simulink library "SatDyn"  (R2018a)
settings: Solver=ode45  StartTime=0.0  StopTime=10.0  RelTol=1e-3
undefined symbols (not defined in the file): ConfParam
settings Model: Creator=y.akisheva  LastModifiedBy=Cédric
settings DataIOCC: LimitDataPoints=on  SaveFormat=Array
settings OptimizationCC: BlockReduction=off  BooleanDataType=off  LifeSpan=inf
settings DebuggingCC: SaveWithParameterizedLinksMsg=none  UnderspecifiedInitializationDetection=Classic  MergeDetectMultiDrivingBlocksExec=none  SignalResolutionControl=TryResolveAllWithWarning  SFUnexpectedBacktrackingDiag=warning  SFNoUnconditionalDefaultTransitionDiag=warning  SFExecutionAtInitializationDiag=none
settings HardwareCC: ProdBitPerPointer=32  ProdBitPerSizeT=32  ProdBitPerPtrDiffT=32  ProdLargestAtomicFloat=None  ProdIntDivRoundTo=Undefined  ProdEndianess=Unspecified  ProdWordSize=32  ProdHWDeviceType=32-bit Generic  TargetUnknown=on
settings ModelReferenceCC: PropagateSignalLabelsOutOfModel=off
settings CodeAppCC: StateflowObjectComments=on
settings GRTTargetCC: TargetLangStandard=C89/C90 (ANSI)  GeneratePreprocessorConditionals=Disable all
settings ConfigComp: CovMetricSettings=dw  CovHtmlReporting=on  CovSaveCumulativeToWorkspaceVar=on  CovSaveSingleToWorkspaceVar=on  CovExternalEMLEnable=off  CovSFcnEnable=off

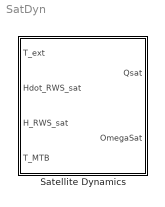
== system SatDyn ==
  Satellite Dynamics : Subsystem

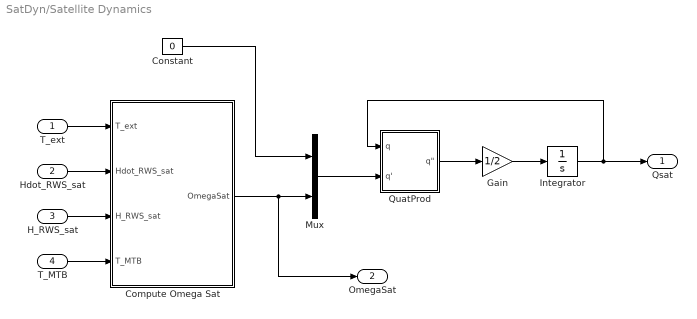
== system SatDyn/Satellite Dynamics ==
  T_ext : Inport
  Hdot_RWS_sat : Inport  Port=2
  H_RWS_sat : Inport  Port=3
  T_MTB : Inport  Port=4
  Compute Omega Sat : Subsystem
  Constant : Constant  Value=0
  Gain : Gain  Gain=1/2
  Integrator : Integrator  InitialCondition=ConfParam.confSatDyn.InitQsat
  Mux : Mux  Inputs=2
  QuatProd : Subsystem  TreatAsAtomicUnit=on
      settings: RTWFcnNameOpts=Use subsystem name  RTWFileNameOpts=Use subsystem name
  Qsat : Outport
  OmegaSat : Outport  Port=2
  wires:
  T_ext/1 -> Compute Omega Sat/1(T_ext)
  Compute Omega Sat/1(OmegaSat) -> OmegaSat/1, Mux/2
  Mux/1 -> QuatProd/2(q')
  Integrator/1 -> Qsat/1, QuatProd/1(q)
  Gain/1 -> Integrator/1
  Hdot_RWS_sat/1 -> Compute Omega Sat/2(Hdot_RWS_sat)
  Constant/1 -> Mux/1
  T_MTB/1 -> Compute Omega Sat/4(T_MTB)
  QuatProd/1("q\"") -> Gain/1
  H_RWS_sat/1 -> Compute Omega Sat/3(H_RWS_sat)

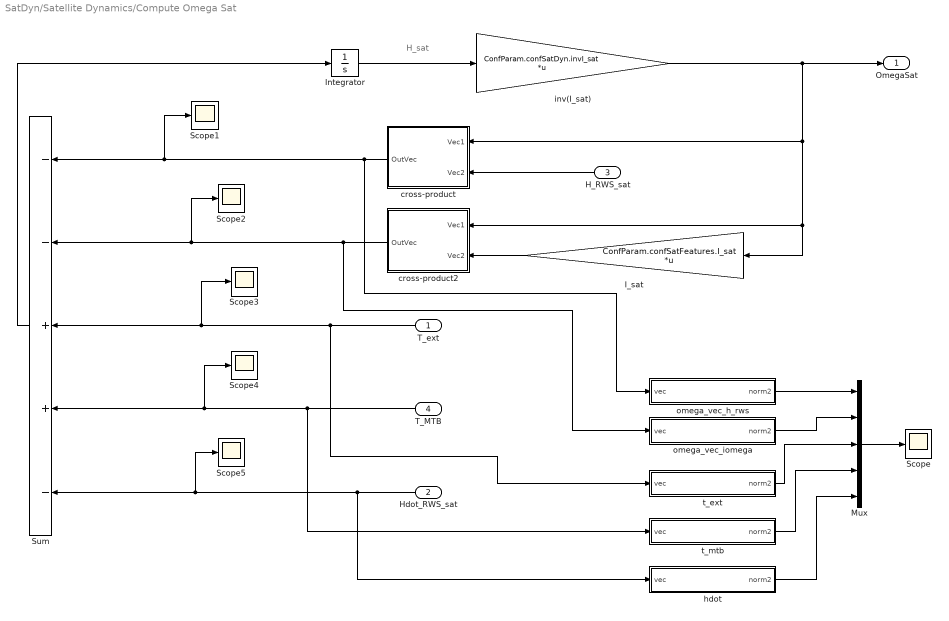
== system SatDyn/Satellite Dynamics/Compute Omega Sat ==
  note: H_sat
  T_ext : Inport
  Hdot_RWS_sat : Inport  Port=2
  H_RWS_sat : Inport  Port=3
  T_MTB : Inport  Port=4
  I_sat : Gain  Gain=ConfParam.confSatFeatures.I_sat  Multiplication=Matrix(K*u)
  Integrator : Integrator  InitialCondition=ConfParam.confSatFeatures.I_sat*ConfParam.confSatDyn.InitOmega_sat
  Mux : Mux  Inputs=5
  Scope{,1..5} (6 alike) : Scope
  Sum : Sum  Inputs=--++-
  cross-product : Subsystem
  cross-product2 : Subsystem
  hdot : Subsystem
  inv(I_sat) : Gain  Gain=ConfParam.confSatDyn.invI_sat  Multiplication=Matrix(K*u)
  omega_vec_h_rws : Subsystem
  omega_vec_iomega : Subsystem
  t_ext : Subsystem
  t_mtb : Subsystem
  OmegaSat : Outport
  wires:
  Hdot_RWS_sat/1 -> hdot/1(vec), Sum/5, Scope5/1
  cross-product/1(OutVec) -> omega_vec_h_rws/1(vec), Sum/1, Scope1/1
  cross-product2/1(OutVec) -> omega_vec_iomega/1(vec), Sum/2, Scope2/1
  omega_vec_h_rws/1(norm2) -> Mux/1
  omega_vec_iomega/1(norm2) -> Mux/2
  t_ext/1(norm2) -> Mux/3
  t_mtb/1(norm2) -> Mux/4
  hdot/1(norm2) -> Mux/5
  Integrator/1 -> inv(I_sat)/1
  inv(I_sat)/1 -> cross-product/1(Vec1), cross-product2/1(Vec1), I_sat/1, OmegaSat/1
  Sum/1 -> Integrator/1
  T_MTB/1 -> Scope4/1, Sum/4, t_mtb/1(vec)
  T_ext/1 -> Sum/3, Scope3/1, t_ext/1(vec)
  I_sat/1 -> cross-product2/2(Vec2)
  H_RWS_sat/1 -> cross-product/2(Vec2)
  Mux/1 -> Scope/1

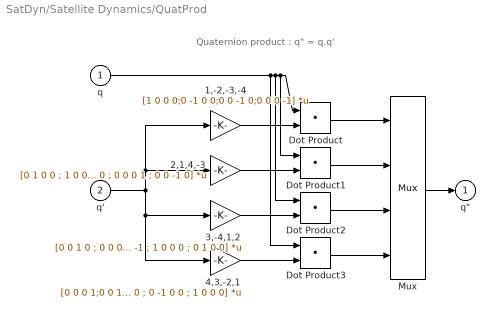
== system SatDyn/Satellite Dynamics/QuatProd ==
  note: Quaternion product : q" = q.q'
  q : Inport  OutDataTypeStr=double  PortDimensions=4
  q' : Inport  Port=2  OutDataTypeStr=double  PortDimensions=4
  1,-2,-3,-4 : Gain  Gain=[1 0 0 0;0 -1 0 0;0 0 -1 0;0 0 0 -1]  Multiplication=Matrix(K*u) (u vector)  SaturateOnIntegerOverflow=on  OutDataTypeStr=Inherit: Same as input  ParamDataTypeStr=Inherit: Same as input
  2,1,4,-3 : Gain  Gain=[0 1 0 0 ; 1 0 0 0 ; 0 0 0 1 ; 0 0 -1 0]  Multiplication=Matrix(K*u) (u vector)  SaturateOnIntegerOverflow=on  OutDataTypeStr=Inherit: Same as input  ParamDataTypeStr=Inherit: Same as input
  3,-4,1,2 : Gain  Gain=[0 0 1 0 ; 0 0 0 -1 ; 1 0 0 0 ; 0 1 0 0]  Multiplication=Matrix(K*u) (u vector)  SaturateOnIntegerOverflow=on  OutDataTypeStr=Inherit: Same as input  ParamDataTypeStr=Inherit: Same as input
  4,3,-2,1 : Gain  Gain=[0 0 0 1;0 0 1 0 ; 0 -1 0 0 ; 1 0 0 0]  Multiplication=Matrix(K*u) (u vector)  SaturateOnIntegerOverflow=on  OutDataTypeStr=Inherit: Same as input  ParamDataTypeStr=Inherit: Same as input
  Dot Product{,1..3} (4 alike) : DotProduct  InputSameDT=on  OutDataTypeStr=Inherit: Inherit via internal rule
  Mux : Mux
  "q\"" : Outport  OutDataTypeStr=double  PortDimensions=4  InitialOutput=0
  wires:
  q'/1 -> 3,-4,1,2/1, 4,3,-2,1/1, 1,-2,-3,-4/1, 2,1,4,-3/1
  1,-2,-3,-4/1 -> Dot Product/2
  2,1,4,-3/1 -> Dot Product1/2
  3,-4,1,2/1 -> Dot Product2/2
  4,3,-2,1/1 -> Dot Product3/2
  q/1 -> Dot Product/1, Dot Product1/1, Dot Product2/1, Dot Product3/1
  Dot Product/1 -> Mux/1
  Dot Product1/1 -> Mux/2
  Dot Product2/1 -> Mux/3
  Dot Product3/1 -> Mux/4
  Mux/1 -> "q\""/1

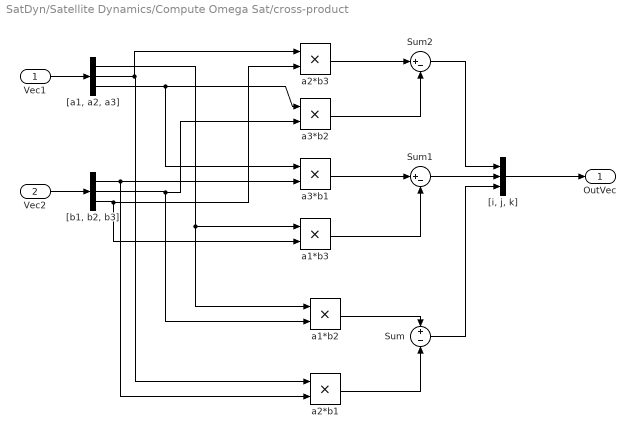
== system SatDyn/Satellite Dynamics/Compute Omega Sat/cross-product ==
  Vec1 : Inport
  Vec2 : Inport  Port=2
  Sum : Sum  Inputs=+-
  Sum1 : Sum  Inputs=|+-
  Sum2 : Sum  Inputs=|+-
  "[a1, a2, a3]" : Demux  Outputs=3
  "[b1, b2, b3]" : Demux  Outputs=3
  "[i, j, k]" : Mux  Inputs=3
  a1*b2 : Product
  a1*b3 : Product
  a2*b1 : Product
  a2*b3 : Product
  a3*b1 : Product
  a3*b2 : Product
  OutVec : Outport
  wires:
  a2*b1/1 -> Sum/2
  "[b1, b2, b3]"/1 -> a3*b1/2, a2*b1/2
  "[a1, a2, a3]"/2 -> a2*b3/1, a2*b1/1
  Vec2/1 -> "[b1, b2, b3]"/1
  "[a1, a2, a3]"/1 -> a1*b3/1, a1*b2/1
  Vec1/1 -> "[a1, a2, a3]"/1
  "[b1, b2, b3]"/2 -> a3*b2/2, a1*b2/2
  a1*b2/1 -> Sum/1
  a3*b1/1 -> Sum1/1
  "[a1, a2, a3]"/3 -> a3*b1/1, a3*b2/1
  a2*b3/1 -> Sum2/1
  "[b1, b2, b3]"/3 -> a2*b3/2, a1*b3/2
  a1*b3/1 -> Sum1/2
  "[i, j, k]"/1 -> OutVec/1
  a3*b2/1 -> Sum2/2
  Sum/1 -> "[i, j, k]"/3
  Sum2/1 -> "[i, j, k]"/1
  Sum1/1 -> "[i, j, k]"/2

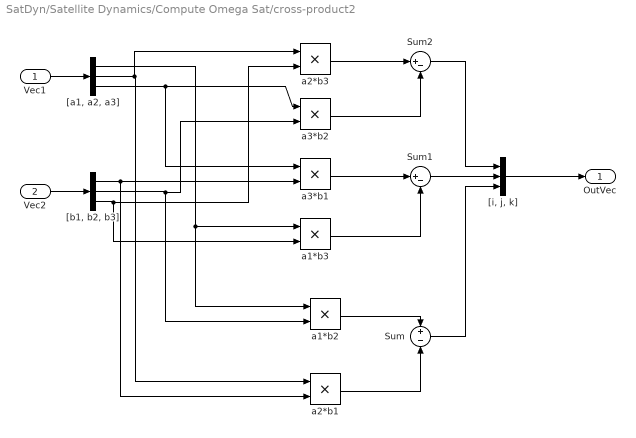
== system SatDyn/Satellite Dynamics/Compute Omega Sat/cross-product2 ==
  Vec1 : Inport
  Vec2 : Inport  Port=2
  Sum : Sum  Inputs=+-
  Sum1 : Sum  Inputs=|+-
  Sum2 : Sum  Inputs=|+-
  "[a1, a2, a3]" : Demux  Outputs=3
  "[b1, b2, b3]" : Demux  Outputs=3
  "[i, j, k]" : Mux  Inputs=3
  a1*b2 : Product
  a1*b3 : Product
  a2*b1 : Product
  a2*b3 : Product
  a3*b1 : Product
  a3*b2 : Product
  OutVec : Outport
  wires:
  a2*b1/1 -> Sum/2
  "[b1, b2, b3]"/1 -> a3*b1/2, a2*b1/2
  "[a1, a2, a3]"/2 -> a2*b3/1, a2*b1/1
  Vec2/1 -> "[b1, b2, b3]"/1
  "[a1, a2, a3]"/1 -> a1*b3/1, a1*b2/1
  Vec1/1 -> "[a1, a2, a3]"/1
  "[b1, b2, b3]"/2 -> a3*b2/2, a1*b2/2
  a1*b2/1 -> Sum/1
  a3*b1/1 -> Sum1/1
  "[a1, a2, a3]"/3 -> a3*b1/1, a3*b2/1
  a2*b3/1 -> Sum2/1
  "[b1, b2, b3]"/3 -> a2*b3/2, a1*b3/2
  a1*b3/1 -> Sum1/2
  "[i, j, k]"/1 -> OutVec/1
  a3*b2/1 -> Sum2/2
  Sum/1 -> "[i, j, k]"/3
  Sum2/1 -> "[i, j, k]"/1
  Sum1/1 -> "[i, j, k]"/2

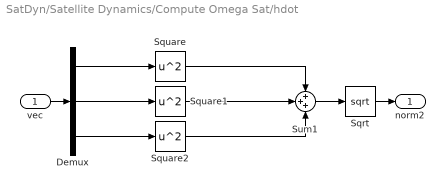
== system SatDyn/Satellite Dynamics/Compute Omega Sat/hdot ==
  vec : Inport
  Demux : Demux  Outputs=3
  Sqrt : Sqrt  SaturateOnIntegerOverflow=on
  Square : Math  Operator=square  SaturateOnIntegerOverflow=on
  Square1 : Math  Operator=square  SaturateOnIntegerOverflow=on
  Square2 : Math  Operator=square  SaturateOnIntegerOverflow=on
  Sum1 : Sum  Inputs=3
  norm2 : Outport
  wires:
  Sum1/1 -> Sqrt/1
  Demux/1 -> Square/1
  Square1/1 -> Sum1/2
  Square2/1 -> Sum1/3
  Demux/3 -> Square2/1
  Square/1 -> Sum1/1
  Demux/2 -> Square1/1
  Sqrt/1 -> norm2/1
  vec/1 -> Demux/1

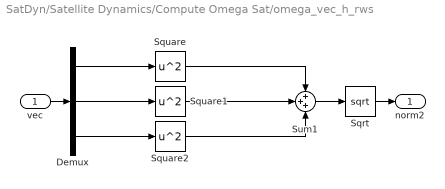
== system SatDyn/Satellite Dynamics/Compute Omega Sat/omega_vec_h_rws ==
  vec : Inport
  Demux : Demux  Outputs=3
  Sqrt : Sqrt  SaturateOnIntegerOverflow=on
  Square : Math  Operator=square  SaturateOnIntegerOverflow=on
  Square1 : Math  Operator=square  SaturateOnIntegerOverflow=on
  Square2 : Math  Operator=square  SaturateOnIntegerOverflow=on
  Sum1 : Sum  Inputs=3
  norm2 : Outport
  wires:
  Sum1/1 -> Sqrt/1
  Demux/1 -> Square/1
  Square1/1 -> Sum1/2
  Square2/1 -> Sum1/3
  Demux/3 -> Square2/1
  Square/1 -> Sum1/1
  Demux/2 -> Square1/1
  Sqrt/1 -> norm2/1
  vec/1 -> Demux/1

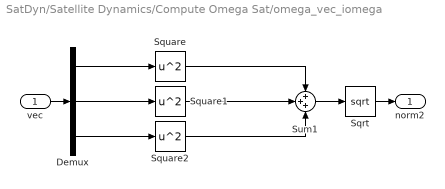
== system SatDyn/Satellite Dynamics/Compute Omega Sat/omega_vec_iomega ==
  vec : Inport
  Demux : Demux  Outputs=3
  Sqrt : Sqrt  SaturateOnIntegerOverflow=on
  Square : Math  Operator=square  SaturateOnIntegerOverflow=on
  Square1 : Math  Operator=square  SaturateOnIntegerOverflow=on
  Square2 : Math  Operator=square  SaturateOnIntegerOverflow=on
  Sum1 : Sum  Inputs=3
  norm2 : Outport
  wires:
  Sum1/1 -> Sqrt/1
  Demux/1 -> Square/1
  Square1/1 -> Sum1/2
  Square2/1 -> Sum1/3
  Demux/3 -> Square2/1
  Square/1 -> Sum1/1
  Demux/2 -> Square1/1
  Sqrt/1 -> norm2/1
  vec/1 -> Demux/1

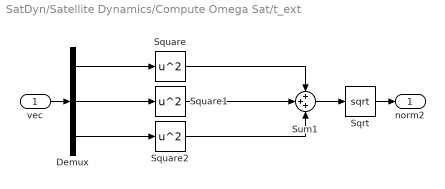
== system SatDyn/Satellite Dynamics/Compute Omega Sat/t_ext ==
  vec : Inport
  Demux : Demux  Outputs=3
  Sqrt : Sqrt  SaturateOnIntegerOverflow=on
  Square : Math  Operator=square  SaturateOnIntegerOverflow=on
  Square1 : Math  Operator=square  SaturateOnIntegerOverflow=on
  Square2 : Math  Operator=square  SaturateOnIntegerOverflow=on
  Sum1 : Sum  Inputs=3
  norm2 : Outport
  wires:
  Sum1/1 -> Sqrt/1
  Demux/1 -> Square/1
  Square1/1 -> Sum1/2
  Square2/1 -> Sum1/3
  Demux/3 -> Square2/1
  Square/1 -> Sum1/1
  Demux/2 -> Square1/1
  Sqrt/1 -> norm2/1
  vec/1 -> Demux/1

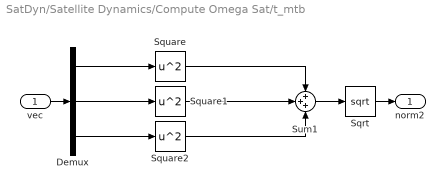
== system SatDyn/Satellite Dynamics/Compute Omega Sat/t_mtb ==
  vec : Inport
  Demux : Demux  Outputs=3
  Sqrt : Sqrt  SaturateOnIntegerOverflow=on
  Square : Math  Operator=square  SaturateOnIntegerOverflow=on
  Square1 : Math  Operator=square  SaturateOnIntegerOverflow=on
  Square2 : Math  Operator=square  SaturateOnIntegerOverflow=on
  Sum1 : Sum  Inputs=3
  norm2 : Outport
  wires:
  Sum1/1 -> Sqrt/1
  Demux/1 -> Square/1
  Square1/1 -> Sum1/2
  Square2/1 -> Sum1/3
  Demux/3 -> Square2/1
  Square/1 -> Sum1/1
  Demux/2 -> Square1/1
  Sqrt/1 -> norm2/1
  vec/1 -> Demux/1
